simulink model "Question2"  (R2022a)
settings: Solver=FixedStepAuto  StartTime=0.0  StopTime=25  FixedStep=1e-4  RelTol=1e-3
settings Model: Creator=Goktug  LastModifiedBy=Goktug

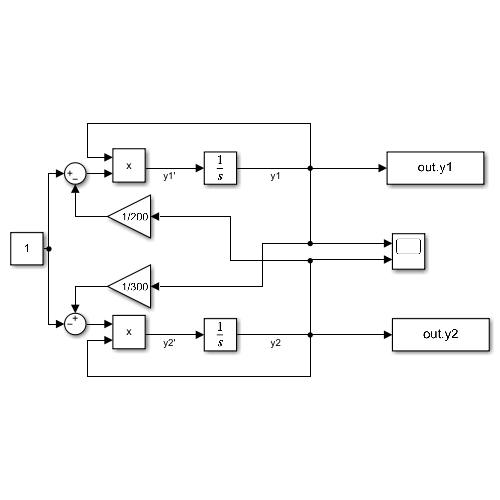
[thumbnail: Simulink's stored preview of the top-level diagram]
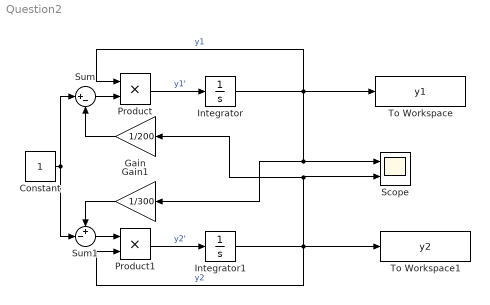
== system Question2 ==
  Constant : Constant
  Gain : Gain  Gain=1/200
  Gain1 : Gain  Gain=1/300
  Integrator : Integrator  InitialCondition=400
  Integrator1 : Integrator  InitialCondition=100
  Product : Product
  Product1 : Product
  Scope : Scope  NumInputPorts=2
  Sum : Sum  Inputs=|+-
  Sum1 : Sum  Inputs=+-|
  To Workspace : ToWorkspace  VariableName=y1  SaveFormat=Timeseries  SampleTime=-1
  To Workspace1 : ToWorkspace  VariableName=y2  SaveFormat=Timeseries  SampleTime=-1
  wires:
  Integrator/1 -> Product/1, Scope/1, Gain1/1, To Workspace/1  "y1"
  Integrator1/1 -> Gain/1, Scope/2, Product1/2, To Workspace1/1  "y2"
  Product/1 -> Integrator/1  "y1'"
  Product1/1 -> Integrator1/1  "y2'"
  Sum/1 -> Product/2
  Gain/1 -> Sum/2
  Sum1/1 -> Product1/1
  Constant/1 -> Sum1/2, Sum/1
  Gain1/1 -> Sum1/1
